simulink model "ars1_project4_Yiwen_ZHANG_Yunfei_ZHAO"  (R2017b)
settings: Solver=VariableStepAuto  StartTime=0.0  StopTime=50  RelTol=1e-3
values from neighbouring files (symbols this model uses):
  A4 = [-1,0,0,0,0,0,0,0,0,0 ... (first row only)    [param.m]
  A5 = [-2,0,0,0,0,0,0,0,1,0 ... (first row only)    [param.m]
  A_C = [0,0,0,0,0,0,0,0,0,0 ... (first row only)    [param.m]
  D1_4 = [d1(1,1) ... (first row only)    [param.m]
  D1_5 = [(d1(1,1)-d1(5,1))+d1(1,1) ... (first row only)    [param.m]
  D2_4 = [d2(1,1) ... (first row only)    [param.m]
  D2_5 = [(d2(1,1)-d2(5,1))+d2(1,1) ... (first row only)    [param.m]
  D_C = [v ... (first row only)    [param.m]
  K1 = 1    [param.m]
  K20 = 20    [param.m]
  K5 = 5    [param.m]
  start = [0;1.5;0;-1.5;-3;3;-3;0;-3;-3]    [param.m]
settings Model: Creator=yunfei  LastModifiedBy=yunfei

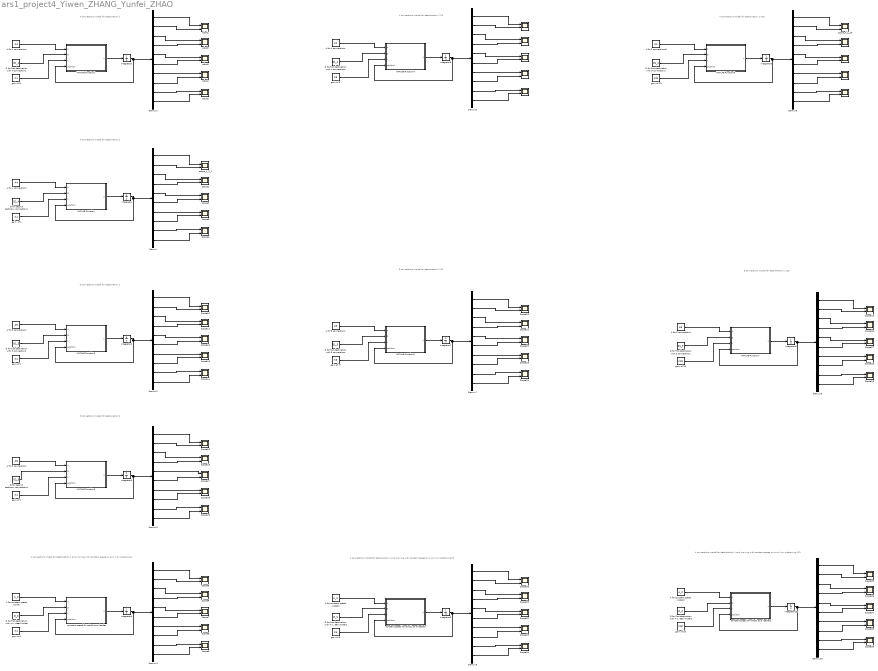
== system ars1_project4_Yiwen_ZHANG_Yunfei_ZHAO ==
  note: 4 connections model for destionation 1
  note: 4 connections model for destionation 2
  note: 5 connections model for destionation 1
  note: 5 connections model for destionation 2
  note: 4 connections model for destionation 1 and moving with constant speed on axis X on platooning
  note: 4 connections model for destionation 1 K5
  note: 4 connections model for destionation 1 K20
  note: 5 connections model for destionation 1 K5
  note: 5 connections model for destionation 1 K20
  note: 4 connections model for destionation 1 and moving with constant speed on axis X on platooning k5
  note: 4 connections model for destionation 1 and moving with constant speed on axis X on platooning K20
  " " : Scope  NumInputPorts=2
  "  " : Scope  NumInputPorts=2
  "   " : Scope  NumInputPorts=2
  "    " : Scope  NumInputPorts=2
  "     " : Scope  NumInputPorts=2
  "        " : Scope  NumInputPorts=2
  "          " : Scope  NumInputPorts=2
  "           " : Scope  NumInputPorts=2
  "             " : Scope  NumInputPorts=2
  " gain of 1 " : Constant  Value=K1
  A for 4 connections : Constant  Value=A4
  "A for 4 connections " : Constant  Value=A4
  "A for 4 connections   " : Constant  Value=A4
  A for 5 connections : Constant  Value=A5
  "A for 5 connections  " : Constant  Value=A5
  "A for 5 connections   " : Constant  Value=A5
  "A for 5 connections    " : Constant  Value=A5
  A for 5 connections5 : Constant  Value=A4
  A for constant speed model : Constant  Value=A_C
  A for constant speed model1 : Constant  Value=A_C
  A for constant speed model2 : Constant  Value=A_C
  D for fisrt destination with 4 connection constant speed model : Constant  Value=D_C
  D for fisrt destination with 4 connection constant speed model1 : Constant  Value=D_C
  D for fisrt destination with 4 connection constant speed model2 : Constant  Value=D_C
  "D for fisrt destination with 4 connections      " : Constant  Value=D1_4
  "D for fisrt destination with 4 connections       " : Constant  Value=D1_4
  "D for fisrt destination with 5 connections " : Constant  Value=D1_5
  "D for fisrt destination with 5 connections  " : Constant  Value=D1_5
  "D for fisrt destination with 5 connections   " : Constant  Value=D1_5
  "D for fisrt destination with 5 connections    " : Constant  Value=D1_4
  "D for second destination with 4 connections " : Constant  Value=D2_4
  "D for second destination with 5 connections     " : Constant  Value=D2_5
  Demux{,1..10} (11 alike) : Demux  Outputs=10
  Integrator{,1..10} (11 alike) : Integrator  InitialCondition=start
  MATLAB Function : MATLAB Function  TreatAsAtomicUnit=on
  MATLAB Function1 : MATLAB Function  TreatAsAtomicUnit=on
  MATLAB Function2 : MATLAB Function  TreatAsAtomicUnit=on
  MATLAB Function3 : MATLAB Function  TreatAsAtomicUnit=on
  MATLAB Function4 : MATLAB Function  TreatAsAtomicUnit=on
  MATLAB Function5 : MATLAB Function  TreatAsAtomicUnit=on
  MATLAB Function6 : MATLAB Function  TreatAsAtomicUnit=on
  MATLAB Function7 : MATLAB Function  TreatAsAtomicUnit=on
  Scope{1..39} (39 alike) : Scope  NumInputPorts=2
  constant speed for robot1 as a leader : MATLAB Function  TreatAsAtomicUnit=on
  constant speed for robot1 as a leader1 : MATLAB Function  TreatAsAtomicUnit=on
  constant speed for robot1 as a leader2 : MATLAB Function  TreatAsAtomicUnit=on
  "gain  of 1 " : Constant  Value=K1
  gain of  5 : Constant  Value=K5
  gain of 1 : Constant  Value=K1
  "gain of 1 " : Constant  Value=K1
  "gain of 1   " : Constant  Value=K1
  gain of 20 : Constant  Value=K20
  "gain of 20 " : Constant  Value=K20
  "gain of 20  " : Constant  Value=K20
  gain of 5 : Constant  Value=K5
  "gain of 5  " : Constant  Value=K5
  robot{1..5} (5 alike) : Scope  NumInputPorts=2
  scope_4_1_20 : Scope  NumInputPorts=2
  scope_4_2_1 : Scope  NumInputPorts=2
  wires:
  Demux1/6 -> robot3/2
  MATLAB Function1/1(u) -> Integrator1/1
  "gain of 1 "/1 -> MATLAB Function1/3(k)
  Demux1/2 -> robot1/2
  Demux1/4 -> robot2/2
  Demux1/10 -> robot5/2
  Demux1/8 -> robot4/2
  Demux1/7 -> robot4/1
  Demux1/3 -> robot2/1
  "A for 4 connections   "/1 -> MATLAB Function1/1(A)
  Demux1/9 -> robot5/1
  Demux1/5 -> robot3/1
  "D for fisrt destination with 4 connections       "/1 -> MATLAB Function1/2(D)
  Demux1/1 -> robot1/1
  Integrator1/1 -> MATLAB Function1/4(position), Demux1/1
  Demux/3 -> Scope1/1
  Demux/2 -> scope_4_2_1/2
  Demux/8 -> Scope3/2
  "gain  of 1 "/1 -> MATLAB Function/3(k)
  Demux/9 -> Scope4/1
  Demux/10 -> Scope4/2
  Demux/4 -> Scope1/2
  A for 4 connections/1 -> MATLAB Function/1(A)
  MATLAB Function/1(u) -> Integrator/1
  Demux/7 -> Scope3/1
  "D for second destination with 4 connections "/1 -> MATLAB Function/2(D)
  Demux/5 -> Scope2/1
  Demux/6 -> Scope2/2
  Integrator/1 -> MATLAB Function/4(position), Demux/1
  Demux/1 -> scope_4_2_1/1
  Demux2/2 -> Scope10/2
  Integrator2/1 -> MATLAB Function2/4(position), Demux2/1
  Demux2/6 -> Scope12/2
  MATLAB Function2/1(u) -> Integrator2/1
  Demux2/1 -> Scope10/1
  "gain of 1   "/1 -> MATLAB Function2/3(k)
  A for 5 connections/1 -> MATLAB Function2/1(A)
  Demux2/4 -> Scope11/2
  Demux2/5 -> Scope12/1
  Demux2/8 -> Scope13/2
  Demux2/9 -> Scope14/1
  Demux2/3 -> Scope11/1
  Demux2/7 -> Scope13/1
  "D for fisrt destination with 5 connections "/1 -> MATLAB Function2/2(D)
  Demux2/10 -> Scope14/2
  " gain of 1 "/1 -> MATLAB Function3/3(k)
  Demux3/4 -> Scope16/2
  Demux3/9 -> Scope19/1
  Demux3/1 -> Scope15/1
  MATLAB Function3/1(u) -> Integrator3/1
  Demux3/7 -> Scope18/1
  Demux3/8 -> Scope18/2
  "A for 5 connections    "/1 -> MATLAB Function3/1(A)
  Demux3/3 -> Scope16/1
  Integrator3/1 -> MATLAB Function3/4(position), Demux3/1
  "D for second destination with 5 connections     "/1 -> MATLAB Function3/2(D)
  Demux3/6 -> Scope17/2
  Demux3/10 -> Scope19/2
  Demux3/2 -> Scope15/2
  Demux3/5 -> Scope17/1
  Demux4/1 -> Scope5/1
  Demux4/2 -> Scope5/2
  Demux4/4 -> Scope6/2
  Demux4/3 -> Scope6/1
  Integrator4/1 -> constant speed for robot1 as a leader/4(position), Demux4/1
  Demux4/7 -> Scope8/1
  constant speed for robot1 as a leader/1(u) -> Integrator4/1
  D for fisrt destination with 4 connection constant speed model/1 -> constant speed for robot1 as a leader/2(D)
  Demux4/9 -> Scope9/1
  Demux4/5 -> Scope7/1
  A for constant speed model/1 -> constant speed for robot1 as a leader/1(A)
  gain of 1/1 -> constant speed for robot1 as a leader/3(k)
  Demux4/6 -> Scope7/2
  Demux4/8 -> Scope8/2
  Demux4/10 -> Scope9/2
  Demux5/4 -> "  "/2
  Demux5/5 -> "   "/1
  Demux5/10 -> "     "/2
  Demux5/8 -> "    "/2
  Demux5/1 -> " "/1
  Demux5/3 -> "  "/1
  Demux5/9 -> "     "/1
  "D for fisrt destination with 4 connections      "/1 -> MATLAB Function4/2(D)
  Demux5/2 -> " "/2
  Integrator5/1 -> MATLAB Function4/4(position), Demux5/1
  Demux5/6 -> "   "/2
  "A for 4 connections "/1 -> MATLAB Function4/1(A)
  Demux5/7 -> "    "/1
  MATLAB Function4/1(u) -> Integrator5/1
  gain of 5/1 -> MATLAB Function4/3(k)
  Demux6/4 -> "        "/2
  Demux6/5 -> "          "/1
  Demux6/10 -> "             "/2
  Demux6/8 -> "           "/2
  Demux6/1 -> scope_4_1_20/1
  Demux6/3 -> "        "/1
  Demux6/9 -> "             "/1
  "D for fisrt destination with 5 connections    "/1 -> MATLAB Function5/2(D)
  Demux6/2 -> scope_4_1_20/2
  Integrator6/1 -> MATLAB Function5/4(position), Demux6/1
  Demux6/6 -> "          "/2
  A for 5 connections5/1 -> MATLAB Function5/1(A)
  Demux6/7 -> "           "/1
  MATLAB Function5/1(u) -> Integrator6/1
  gain of 20/1 -> MATLAB Function5/3(k)
  Integrator7/1 -> MATLAB Function6/4(position), Demux7/1
  Demux7/7 -> Scope23/1
  Demux7/9 -> Scope24/1
  Demux7/3 -> Scope21/1
  Demux7/4 -> Scope21/2
  MATLAB Function6/1(u) -> Integrator7/1
  Demux7/10 -> Scope24/2
  Demux7/6 -> Scope22/2
  "D for fisrt destination with 5 connections   "/1 -> MATLAB Function6/2(D)
  Demux7/8 -> Scope23/2
  gain of  5/1 -> MATLAB Function6/3(k)
  Demux7/1 -> Scope20/1
  Demux7/2 -> Scope20/2
  Demux7/5 -> Scope22/1
  "A for 5 connections  "/1 -> MATLAB Function6/1(A)
  Integrator8/1 -> MATLAB Function7/4(position), Demux8/1
  Demux8/7 -> Scope28/1
  Demux8/9 -> Scope29/1
  Demux8/3 -> Scope26/1
  Demux8/4 -> Scope26/2
  MATLAB Function7/1(u) -> Integrator8/1
  Demux8/10 -> Scope29/2
  Demux8/6 -> Scope27/2
  "D for fisrt destination with 5 connections  "/1 -> MATLAB Function7/2(D)
  Demux8/8 -> Scope28/2
  "gain of 20 "/1 -> MATLAB Function7/3(k)
  Demux8/1 -> Scope25/1
  Demux8/2 -> Scope25/2
  Demux8/5 -> Scope27/1
  "A for 5 connections   "/1 -> MATLAB Function7/1(A)
  Demux9/4 -> Scope31/2
  constant speed for robot1 as a leader1/1(u) -> Integrator9/1
  A for constant speed model1/1 -> constant speed for robot1 as a leader1/1(A)
  Demux9/7 -> Scope33/1
  Integrator9/1 -> constant speed for robot1 as a leader1/4(position), Demux9/1
  Demux9/5 -> Scope32/1
  Demux9/1 -> Scope30/1
  Demux9/3 -> Scope31/1
  Demux9/2 -> Scope30/2
  Demux9/9 -> Scope34/1
  Demux9/10 -> Scope34/2
  D for fisrt destination with 4 connection constant speed model1/1 -> constant speed for robot1 as a leader1/2(D)
  "gain of 5  "/1 -> constant speed for robot1 as a leader1/3(k)
  Demux9/8 -> Scope33/2
  Demux9/6 -> Scope32/2
  Demux10/4 -> Scope36/2
  constant speed for robot1 as a leader2/1(u) -> Integrator10/1
  A for constant speed model2/1 -> constant speed for robot1 as a leader2/1(A)
  Demux10/7 -> Scope38/1
  Integrator10/1 -> constant speed for robot1 as a leader2/4(position), Demux10/1
  Demux10/5 -> Scope37/1
  Demux10/1 -> Scope35/1
  Demux10/3 -> Scope36/1
  Demux10/2 -> Scope35/2
  Demux10/9 -> Scope39/1
  Demux10/10 -> Scope39/2
  D for fisrt destination with 4 connection constant speed model2/1 -> constant speed for robot1 as a leader2/2(D)
  "gain of 20  "/1 -> constant speed for robot1 as a leader2/3(k)
  Demux10/8 -> Scope38/2
  Demux10/6 -> Scope37/2

== matlab function ars1_project4_Yiwen_ZHANG_Yunfei_ZHAO/MATLAB Function1 ==
  data: A input; u output; D input; k input; position input
function u = fcn(A, D, k, position)
    u = k*(A * position + D);
end

== matlab function ars1_project4_Yiwen_ZHANG_Yunfei_ZHAO/MATLAB Function ==
  data: A input; u output; D input; k input; position input
function u = fcn(A, D, k, position)
    u = k * (A * position + D);
end

== matlab function ars1_project4_Yiwen_ZHANG_Yunfei_ZHAO/MATLAB Function2 ==
  data: A input; u output; D input; k input; position input
function u = fcn(A, D, k, position)
    u = k * (A * position + D);
end

== matlab function ars1_project4_Yiwen_ZHANG_Yunfei_ZHAO/MATLAB Function3 ==
  data: A input; u output; D input; k input; position input
function u = fcn(A, D, k, position)
    u = k * (A * position + D);
end

== matlab function ars1_project4_Yiwen_ZHANG_Yunfei_ZHAO/constant speed for robot1 as a leader ==
  data: A input; u output; D input; k input; position input
function u = fcn(A, D, k, position)
    u = k * (A * position + D);
end

== matlab function ars1_project4_Yiwen_ZHANG_Yunfei_ZHAO/MATLAB Function4 ==
  data: A input; u output; D input; k input; position input
function u = fcn(A, D, k, position)
    u = k*(A * position + D);
end

== matlab function ars1_project4_Yiwen_ZHANG_Yunfei_ZHAO/MATLAB Function5 ==
  data: A input; u output; D input; k input; position input
function u = fcn(A, D, k, position)
    u = k*(A * position + D);
end

== matlab function ars1_project4_Yiwen_ZHANG_Yunfei_ZHAO/MATLAB Function6 ==
  data: A input; u output; D input; k input; position input
function u = fcn(A, D, k, position)
    u = k*(A * position + D);
end

== matlab function ars1_project4_Yiwen_ZHANG_Yunfei_ZHAO/MATLAB Function7 ==
  data: A input; u output; D input; k input; position input
function u = fcn(A, D, k, position)
    u = k * (A * position + D);
end

== matlab function ars1_project4_Yiwen_ZHANG_Yunfei_ZHAO/constant speed for robot1 as a leader1 ==
  data: A input; u output; D input; k input; position input
function u = fcn(A, D, k, position)
    u = k * (A * position + D);
end

== matlab function ars1_project4_Yiwen_ZHANG_Yunfei_ZHAO/constant speed for robot1 as a leader2 ==
  data: A input; u output; D input; k input; position input
function u = fcn(A, D, k, position)
    u = k * (A * position + D);
end
